simulink model "quadtestmodel"  (R2013a)
settings: Solver=ode45  StartTime=0.0  StopTime=10  RelTol=1e-3
undefined symbols (not defined in the file or in its folder): e0_0, e1_0, e2_0, e3_0, m, s
libraries: simulink x4, aerolibtransform2 x3, aerolib6dofsys x2, aerolibconvert2 x2, aerolibutil x1, aerolibanim x1, aerolibnav x1
settings Model: Creator=Oskar  LastModifiedBy=Oskar
settings DataIOCC: SignalLoggingSaveFormat=ModelDataLogs
settings OptimizationCC: ExpressionDepthLimit=2147483647
settings DebuggingCC: FcnCallInpInsideContextMsg=UseLocalSettings
settings SFSimCC: SimParseCustomCode=off
settings GRTTargetCC: CombineOutputUpdateFcns=off  GRTInterface=on

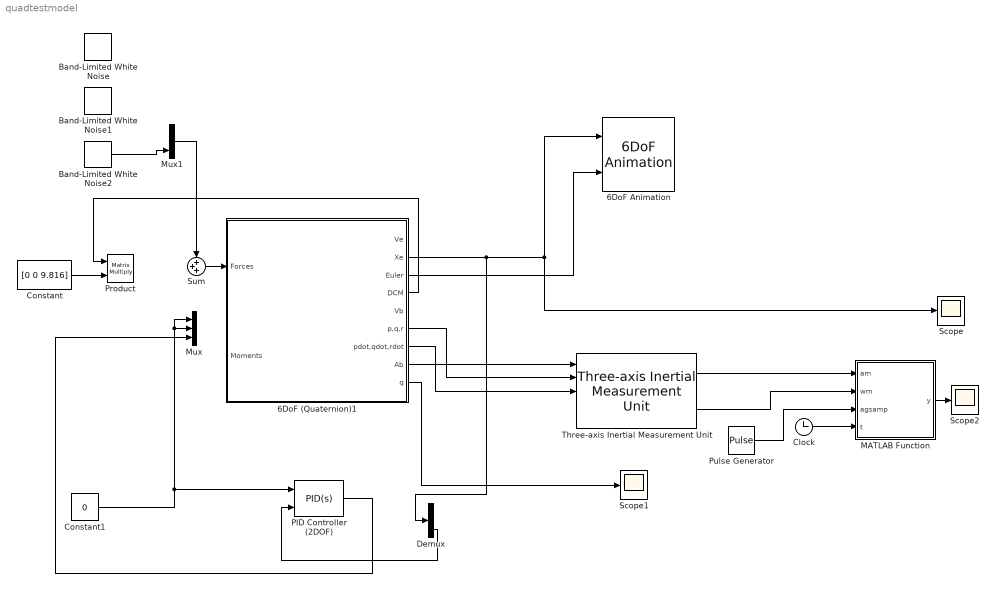
== system quadtestmodel ==
  6DoF (Quaternion)1 : Subsystem  mask(6DoF EoM (Body Axis)){units=Metric (MKS), mtype=Fixed, rep=Quaternion, xme_0=[0 0 0], Vm_0=[0 0 0], eul_0=[0 0 0], pm_0=[0 0 0], mass_0=1.0, mass_e=0, mass_f=0, inertia=eye(3), inertia_e=eye(3), inertia_f=eye(3), k_quat=1.0}
      mask prompts: mtype "Mass type:"; rep "Representation:"; xme_0 "Initial position in inertial axes [Xe,Ye,Ze]:"; Vm_0 "Initial velocity in body axes [U,v,w]:"; eul_0 "Initial Euler orientation [roll, pitch, yaw]:"; pm_0 "Initial body rotation rates [p,q,r]:"; mass_0 "Initial mass:"; mass_e "Empty mass:"; mass_f "Full mass:"; inertia_e "Empty inertia matrix:"; inertia_f "Full inertia matrix:"; k_quat "Gain for quaternion normalization:"
      mask help: Integrate the six-degrees-of-freedom equations of motion in body axis.
      mask init:
      | ports=aeroicon('aeroblk6dofbody','icon');
      mask Help: eval('asbhelp(''sixdof_quaternion'')');
      mask TypeOptions units: Metric (MKS) | English (Velocity in ft/s) | English (Velocity in kts)
      mask TypeOptions mtype: Fixed | Simple Variable | Custom Variable
      mask Callback mtype: aeroicon('aeroblk6dofbody');
      mask TypeOptions rep: Euler Angles | Quaternion
      mask Callback rep: aeroicon('aeroblk6dofbody');
      mask Display:
      | port_label(ports(1).type,ports(1).port,ports(1).txt,'texmode','on');
      | port_label(ports(2).type,ports(2).port,ports(2).txt,'texmode','on');
      | port_label(ports(3).type,ports(3).port,ports(3).txt,'texmode','on');
      | port_label(ports(4).type,ports(4).port,ports(4).txt,'texmode','on');
      | port_label(ports(5).type,ports(5).port,ports(5).txt,'texmode','on');
      | port_label(ports(6).type,ports(6).port,ports(6).txt,'texmode','on');
      | port_label(ports(7).type,ports(7).port,ports(7).txt,'texmode','on');
      | port_label(ports(8).type,ports(8).port,ports(8).txt,'texmode','on');
      | port_label(ports(9).type,ports(9).port,ports(9).txt,'texmode','on');
      | port_label(ports(10).type,ports(10).port,ports(10).txt,'texmode','on');
      | port_label(ports(11).type,ports(11).port,ports(11).txt,'texmode','on');
      | port_label(ports(12).type,ports(12).port,ports(12).txt,'texmode','on');
      | port_label(ports(13).type,ports(13).port,ports(13).txt,'texmode','on');
      | port_label(ports(14).type,ports(14).port,ports(14).txt,'texmode','on');
      | port_label(ports(15).type,ports(15).port,ports(15).txt,'texmode','on');
      | [x y xp yp highstr lowstr maxy miny]=aeroimage('sixdofbody',gcbh);
      | text(0.5,maxy+0.065,highstr{:},'horizontalAlignment','center')
      | text(0.5,miny-0.05,lowstr{:},'horizontalAlignment','center')
      | plot(x,y);
      | patch(xp, yp);
      | port_label('output', 9, 'q');
  6DoF Animation : aerolibanim/6DoF Animation  u1=[-5 5 -5 5 -5 5]  u2=0.1  u3=1.0  u4=[4000 0 -5000]  u5=Fixed position  u6=[12 10 -7]  u7=35  u8=on
  Band-Limited White Noise : simulink/Sources/Band-Limited White Noise  Cov=[0.1]  Ts=0.01  seed=[1339]
  Band-Limited White Noise1 : simulink/Sources/Band-Limited White Noise  Cov=[0.1]  Ts=0.01  seed=[1338]
  Band-Limited White Noise2 : simulink/Sources/Band-Limited White Noise  Cov=[0.1]  Ts=0.01  seed=[1337]
  Clock : Clock
  Constant : Constant  Value=[0 0 9.816]
  Constant1 : Constant  Value=0
  Demux : Demux  Outputs=3
  MATLAB Function : MATLAB Function  TreatAsAtomicUnit=on
  Mux : Mux  Inputs=3
  Mux1 : Mux  Inputs=3
  PID Controller (2DOF) : simulink/Continuous/PID Controller (2DOF)  Controller=PID  TimeDomain=Continuous-time  SampleTime=1  IntegratorMethod=Forward Euler  FilterMethod=Forward Euler  Form=Parallel  P=8.36590741908302  I=0.631118206976681  D=10.1139382064284  N=20.2743419407708  b=1  c=1  InitialConditionSource=internal  InitialConditionForIntegrator=-12  InitialConditionForFilter=0  ExternalReset=none  LimitOutput=off  UpperSaturationLimit=inf  LowerSaturationLimit=-inf  LinearizeAsGain=off  AntiWindupMode=none  Kb=1  TrackingMode=off  Kt=1  PParamMin=[]  PParamMax=[]  IParamMin=[]  IParamMax=[]  DParamMin=[]  DParamMax=[]  NParamMin=[]  NParamMax=[]  bParamMin=[]  bParamMax=[]  cParamMin=[]  cParamMax=[]  KbParamMin=[]  KbParamMax=[]  KtParamMin=[]  KtParamMax=[]  POutMin=[]  POutMax=[]  IOutMin=[]  IOutMax=[]  DOutMin=[]  DOutMax=[]  NOutMin=[]  NOutMax=[]  bOutMin=[]  bOutMax=[]  cOutMin=[]  cOutMax=[]  KbOutMin=[]  KbOutMax=[]  KtOutMin=[]  KtOutMax=[]  IntegratorOutMin=[]  IntegratorOutMax=[]  FilterOutMin=[]  FilterOutMax=[]  SumOutMin=[]  SumOutMax=[]  Sum1OutMin=[]  Sum1OutMax=[]  Sum2OutMin=[]  Sum2OutMax=[]  Sum3OutMin=[]  Sum3OutMax=[]  SumI1OutMin=[]  SumI1OutMax=[]  SumI2OutMin=[]  SumI2OutMax=[]  SumI3OutMin=[]  SumI3OutMax=[]  SumDOutMin=[]  SumDOutMax=[]  SaturationOutMin=[]  SaturationOutMax=[]  IntegratorContinuousStateAttributes=''  IntegratorStateMustResolveToSignalObject=off  IntegratorRTWStateStorageClass=Auto  FilterContinuousStateAttributes=''  FilterStateMustResolveToSignalObject=off  FilterRTWStateStorageClass=Auto
  Product : Product  Multiplication=Matrix(*)  RndMeth=Zero
  Pulse Generator : DiscretePulseGenerator  PulseType=Time based  Period=0.02  PulseWidth=50
  Scope : Scope
      settings: TimeRange=10
  Scope1 : Scope
  Scope2 : Scope
      settings: SaveName=ScopeData2
  Sum : Sum  Inputs=+++
  Three-axis Inertial Measurement Unit : aerolibnav/Three-axis Inertial Measurement Unit  units=Metric (MKS)  imu=[0 0 0]  dtype_a=on  w_a=190  z_a=0.707  a_sf_cc=[1 0 0; 0 1 0; 0 0 1]  a_bias=[0 0 0]  a_sat="[-inf  -inf  -inf  inf inf inf]"  dtype_g=on  w_g=190  z_g=0.707  g_sf_cc=[1 0 0; 0 1 0; 0 0 1]  g_bias=[0 0 0]  g_sens=[0 0 0]  g_sat="[-inf  -inf  -inf  inf inf inf]"  i_rand=on  i_seeds=[23093 23094 23095 23096 23097 23098]  i_pow=[0.001 0.001 0.001 0.0001 0.0001 0.0001]  i_Ts=0
  wires:
  6DoF (Quaternion)1/3(Euler) -> 6DoF Animation/2
  6DoF (Quaternion)1/8(Ab) -> Three-axis Inertial Measurement Unit/1
  6DoF (Quaternion)1/6(p,q,r) -> Three-axis Inertial Measurement Unit/2
  6DoF (Quaternion)1/7(pdot,qdot,rdot) -> Three-axis Inertial Measurement Unit/3
  6DoF (Quaternion)1/4(DCM) -> Product/1
  Constant/1 -> Product/2
  6DoF (Quaternion)1/2(Xe) -> Scope/1, 6DoF Animation/1, Demux/1
  Constant1/1 -> Mux/1, Mux/2, PID Controller (2DOF)/1
  Demux/3 -> PID Controller (2DOF)/2
  Sum/1 -> 6DoF (Quaternion)1/1(Forces)
  6DoF (Quaternion)1/9(q) -> Scope1/1
  PID Controller (2DOF)/1 -> Mux/3
  Three-axis Inertial Measurement Unit/1 -> MATLAB Function/1(am)
  Three-axis Inertial Measurement Unit/2 -> MATLAB Function/2(wm)
  MATLAB Function/1(y) -> Scope2/1
  Pulse Generator/1 -> MATLAB Function/3(agsamp)
  Clock/1 -> MATLAB Function/4(t)
  Mux1/1 -> Sum/1
  Band-Limited White Noise2/1 -> Mux1/3

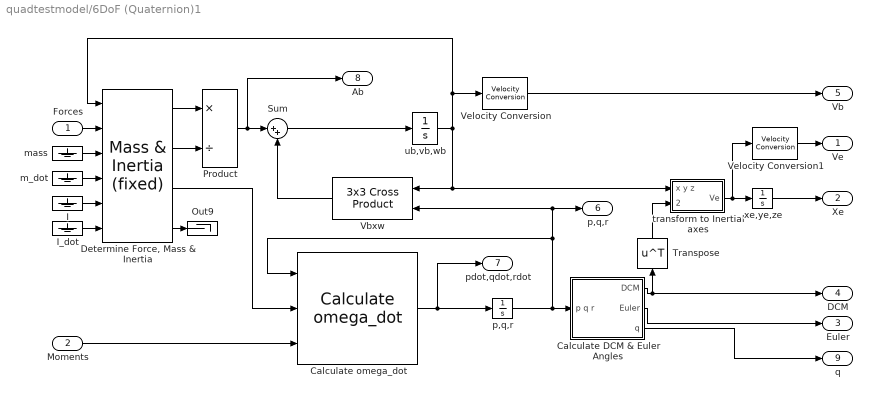
== system quadtestmodel/6DoF (Quaternion)1 ==
  Forces : Inport
  Moments : Inport  Port=2
  Calculate DCM & Euler Angles : Subsystem  AncestorBlock=aerolib6dofsys/DCM & Euler Angles (Quaternion)  mask(DCM & Euler Angles (Quaternion)){}
  Calculate omega_dot : aerolib6dofsys/Calculate omega_dot
  "Determine Force, Mass & Inertia" : aerolib6dofsys/Mass & Inertia (fixed)  SystemSampleTime=-1
  I : Ground
  I_dot : Ground
  Out9 : Terminator
  Product : Product  Inputs=*/  SaturateOnIntegerOverflow=on  OutDataTypeStr=Inherit: Same as first input
  Sum : Sum  Inputs=|++  SaturateOnIntegerOverflow=on
  Transpose : Math  Operator=transpose  SaturateOnIntegerOverflow=on
  Vbxw : aerolibutil/3x3 Cross Product
  Velocity Conversion : aerolibconvert2/Velocity Conversion  IU=m/s  OU=m/s
  Velocity Conversion1 : aerolibconvert2/Velocity Conversion  IU=m/s  OU=m/s
  m_dot : Ground
  mass : Ground
  "p,q,r " : Integrator  InitialCondition=pm_0
  "transform to Inertial axes " : Subsystem  mask(Vector Transformation){}
      mask Display: disp('L_EB')
  ub,vb,wb : Integrator  InitialCondition=convvel(Vm_0,'m/s','m/s')
  xe,ye,ze : Integrator  InitialCondition=xme_0
  Ve : Outport
  Xe : Outport  Port=2
  Euler : Outport  Port=3
  DCM : Outport  Port=4
  Vb : Outport  Port=5
  p,q,r : Outport  Port=6
  pdot,qdot,rdot : Outport  Port=7
  Ab : Outport  Port=8
  q : Outport  Port=9
  wires:
  "Determine Force, Mass & Inertia"/1 -> Product/1
  I_dot/1 -> "Determine Force, Mass & Inertia"/6
  I/1 -> "Determine Force, Mass & Inertia"/5
  Calculate omega_dot/1 -> "p,q,r "/1, pdot,qdot,rdot/1
  "Determine Force, Mass & Inertia"/4 -> Out9/1
  m_dot/1 -> "Determine Force, Mass & Inertia"/4
  "Determine Force, Mass & Inertia"/2 -> Product/2
  mass/1 -> "Determine Force, Mass & Inertia"/3
  Transpose/1 -> "transform to Inertial axes "/2(transform coefficients)
  Calculate DCM & Euler Angles/1(DCM) -> Transpose/1, DCM/1
  Product/1 -> Ab/1, Sum/1
  Forces/1 -> "Determine Force, Mass & Inertia"/2
  Moments/1 -> Calculate omega_dot/3
  "p,q,r "/1 -> Calculate omega_dot/1, Vbxw/2, p,q,r/1, Calculate DCM & Euler Angles/1(p q r)
  "transform to Inertial axes "/1(Ve) -> xe,ye,ze/1, Velocity Conversion1/1
  xe,ye,ze/1 -> Xe/1
  Sum/1 -> ub,vb,wb/1
  ub,vb,wb/1 -> "Determine Force, Mass & Inertia"/1, Velocity Conversion/1, Vbxw/1, "transform to Inertial axes "/1(x y z)
  Vbxw/1 -> Sum/2
  Calculate DCM & Euler Angles/2(Euler) -> Euler/1
  "Determine Force, Mass & Inertia"/3 -> Calculate omega_dot/2
  Velocity Conversion/1 -> Vb/1
  Velocity Conversion1/1 -> Ve/1
  Calculate DCM & Euler Angles/3(q) -> q/1

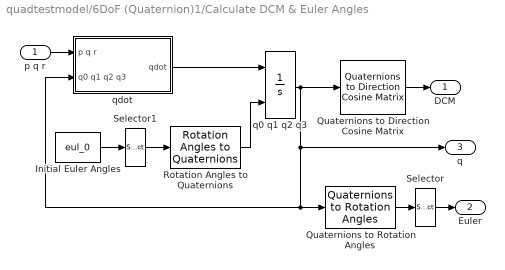
== system quadtestmodel/6DoF (Quaternion)1/Calculate DCM & Euler Angles ==
  p q r : Inport
  Initial Euler Angles : Constant  Value=eul_0
  Quaternions to Direction Cosine Matrix : aerolibtransform2/Quaternions to  Direction Cosine Matrix
  Quaternions to Rotation Angles : aerolibtransform2/Quaternions to Rotation Angles  rotationOrder=ZYX
  Rotation Angles to Quaternions : aerolibtransform2/Rotation Angles to Quaternions  rotationOrder=ZYX
  Selector : Selector  InputPortWidth=3  IndexOptions=Index vector (dialog)  Indices=[3 2 1]  OutputSizes=1
  Selector1 : Selector  InputPortWidth=3  IndexOptions=Index vector (dialog)  Indices=[3 2 1]  OutputSizes=1
  q0 q1 q2 q3 : Integrator  InitialConditionSource=external  InitialCondition=[e0_0 e1_0 e2_0 e3_0]
  qdot : Subsystem
  DCM : Outport
  Euler : Outport  Port=2
  q : Outport  Port=3
  wires:
  Selector1/1 -> Rotation Angles to Quaternions/1
  Selector/1 -> Euler/1
  Quaternions to Rotation Angles/1 -> Selector/1
  Quaternions to Direction Cosine Matrix/1 -> DCM/1
  p q r/1 -> qdot/1(p q r)
  Initial Euler Angles/1 -> Selector1/1
  Rotation Angles to Quaternions/1 -> q0 q1 q2 q3/2
  q0 q1 q2 q3/1 -> Quaternions to Direction Cosine Matrix/1, q/1, Quaternions to Rotation Angles/1, qdot/2(q0 q1 q2 q3)
  qdot/1(qdot) -> q0 q1 q2 q3/1

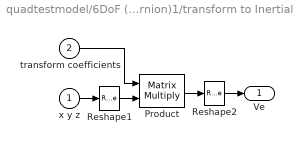
== system quadtestmodel/6DoF (Quaternion)1/transform to Inertial axes  ==
  x y z : Inport
  transform coefficients : Inport  Port=2
  Product : Product  Multiplication=Matrix(*)  SaturateOnIntegerOverflow=on  InputSameDT=on  OutDataTypeStr=Inherit: Same as first input
  Reshape1 : Reshape  OutputDimensionality=Column vector (2-D)
  Reshape2 : Reshape
  Ve : Outport
  wires:
  Reshape2/1 -> Ve/1
  Reshape1/1 -> Product/2
  x y z/1 -> Reshape1/1
  transform coefficients/1 -> Product/1
  Product/1 -> Reshape2/1

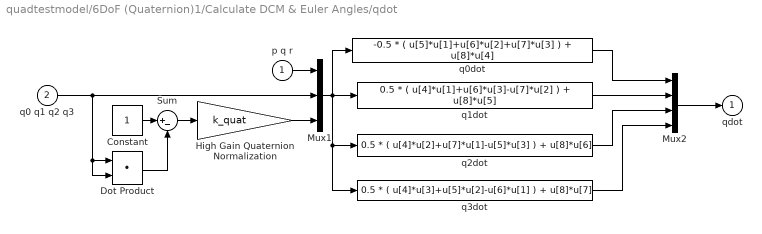
== system quadtestmodel/6DoF (Quaternion)1/Calculate DCM & Euler Angles/qdot ==
  p q r : Inport
  q0 q1 q2 q3 : Inport  Port=2
  Constant : Constant
  Dot Product : DotProduct  OutDataTypeStr=Inherit: Inherit via internal rule
  High Gain Quaternion Normalization : Gain  Gain=k_quat  SaturateOnIntegerOverflow=on  OutDataTypeStr=Inherit: Same as input  ParamDataTypeStr=Inherit: Same as input
  Mux1 : Mux  Inputs=[3 4 1]
  Mux2 : Mux
  Sum : Sum  Inputs=|+-  SaturateOnIntegerOverflow=on  InputSameDT=on  OutDataTypeStr=Inherit: Same as first input
  q0dot : Fcn  Expr=-0.5 * ( u[5]*u[1]+u[6]*u[2]+u[7]*u[3] ) + u[8]*u[4]
  q1dot : Fcn  Expr=0.5 * ( u[4]*u[1]+u[6]*u[3]-u[7]*u[2] ) + u[8]*u[5]
  q2dot : Fcn  Expr=0.5 * ( u[4]*u[2]+u[7]*u[1]-u[5]*u[3] ) + u[8]*u[6]
  q3dot : Fcn  Expr=0.5 * ( u[4]*u[3]+u[5]*u[2]-u[6]*u[1] ) + u[8]*u[7]
  qdot : Outport  InitialOutput=0
  wires:
  p q r/1 -> Mux1/1
  Dot Product/1 -> Sum/2
  High Gain Quaternion Normalization/1 -> Mux1/3
  Sum/1 -> High Gain Quaternion Normalization/1
  Constant/1 -> Sum/1
  Mux2/1 -> qdot/1
  q0dot/1 -> Mux2/1
  q1dot/1 -> Mux2/2
  q2dot/1 -> Mux2/3
  Mux1/1 -> q2dot/1, q3dot/1, q0dot/1, q1dot/1
  q3dot/1 -> Mux2/4
  q0 q1 q2 q3/1 -> Dot Product/1, Dot Product/2, Mux1/2

== matlab function quadtestmodel/MATLAB Function ==
  data: am input; y output; wm input; agsamp input; t input
%Code documentation here please

function y = predict(am, wm, agsamp, t)
%#codegen

persistent P X oldagsamp oldt
if isempty(oldt)
    oldt = 0;
end
if isempty(oldagsamp)
    oldagsamp = 0;
end
if isempty(X)
   X = [[0 0 0]'; [0 0 0]'; [1 0 0 0]'; [0 0 0]'; [0 0 0]']; 
end
if isempty(P)
   P = zeros(16); 
end

Q = [diag([0.0001 0.0001 0.0001 0.001 0.001 0.001 0 0 0 0 0 0])];

Xdot = zeros(16,1);

if agsamp ~= oldagsamp
    oldagsamp = agsamp;
    Ts = t-oldt;
    oldt = t;
    
    w = wm - X(11:13);
    a = am - X(14:16);
    q = X(7:10);
    
    Omega = [0    -w(1) -w(2) -w(3); ...
             w(1)  0     w(3) -w(2); ...
             w(2) -w(3)  0     w(1); ...
             w(3)  w(2) -w(1)  0];
    
    Xi = [-q(2) -q(3) -q(4); ...
           q(1) -q(4)  q(3); ...
           q(4)  q(1) -q(2); ...
          -q(3)  q(2)  q(1)];

    %DCM = quat2dcm(X(7:10));
    %DCMderiv = [norm(q)^2-2*q(3)*q(3)-2*q(4)*q(4) 2*q(2)*q(3)+2*q(4)*q(1) 2*q(2)*q(4)-2*q(3)*q(1);
    %       2*q(2)*q(3)-2*q(4)*q(1) norm(q)^2-2*q(2)*q(2)-2*q(4)*q(4) 2*q(3)*q(4)+2*q(2)*q(1);
    %       2*q(2)*q(4)+2*q(3)*q(1) 2*q(3)*q(4)-2*q(2)*q(1) norm(q)^2-2*q(2)*q(2)-2*q(3)*q(3)];
    
    DCM = [1-2*q(3)*q(3)-2*q(4)*q(4) 2*q(2)*q(3)+2*q(4)*q(1) 2*q(2)*q(4)-2*q(3)*q(1);
           2*q(2)*q(3)-2*q(4)*q(1) 1-2*q(2)*q(2)-2*q(4)*q(4) 2*q(3)*q(4)+2*q(2)*q(1);
           2*q(2)*q(4)+2*q(3)*q(1) 2*q(3)*q(4)-2*q(2)*q(1) 1-2*q(2)*q(2)-2*q(3)*q(3)];
          

    %Transform X
       
    %Pos
    Xdot(1:3) = X(4:6);
    
    %vel
    Xdot(4:6) = DCM.' * a;
    Xdot(6) = Xdot(6) + 0;% 9.816;

    %quat
    Xdot(7:10) = 0.5 .* Xi * w;

    %biases
    Xdot(11:16) = 0;
    
    X = X + Xdot.*Ts;
    X(7:10) = X(7:10)/norm(X(7:10));

    %random stuff about G
    %q = rand(4,1); q = q./norm(q); Xi = [-q(2) -q(3) -q(4); q(1) -q(4) q(3); q(4) q(1) -q(2); -q(3) q(2) q(1)]; 
    %A = [zeros(3,13); [zeros(3)] [orth(rand(3))] [zeros(3,7)]; Xi zeros(4,10); zeros(3,6) eye(3) zeros(3,4)]; A*A'
    
    % Transform P
    
    Fvqparts = Xi * a;
    Fvq = 2 .* [Fvqparts(2) -Fvqparts(1) Fvqparts(4) -Fvqparts(3); ...
                Fvqparts(3) -Fvqparts(4) -Fvqparts(1) Fvqparts(2); ...
                Fvqparts(4) Fvqparts(3) -Fvqparts(2) -Fvqparts(1)];
    
    Fvba = -DCM.';
    Fqq = 0.5 .* Omega;
    Fqbw = -0.5 .* Xi;
    
    F = eye(16) + Ts.* [zeros(3) eye(3) zeros(3, 10); ...
                        zeros(3,6) Fvq zeros(3) Fvba; ...
                        zeros(4,6) Fqq Fqbw zeros(4,3); ...
                        zeros(6,16)];
    
    Gvwa = DCM.';
    Gqww = 0.5 .* Xi;
    
    G = Ts.* [zeros(3, 12); ...
              zeros(3) Gvwa zeros(3,6); ...
              Gqww zeros(4, 9); ...
              zeros(3,6) eye(3) zeros(3); ...
              zeros(3,9) eye(3)];
    
    P = F*P*F.' + G*Q*G.';
    
end

y = X;
